simulink model "sl_subsys_fcncallerr12"  (Simulink 7.6)
settings: Solver=FixedStepDiscrete  StartTime=0.0  StopTime=10.0  FixedStep=1  RelTol=1e-3
libraries: simulink x4
Description:
  | Function-call subsystems whose inputs are directly or indirectly computed during execution of the function-call
  | 
  | In each of the function-call subsystems below, one of the inputs is either directly
  | or indirectly computed during the computation of the function-call subsystems outputs. As
  | a result, one can alter the output values produced by the function-call by subtly affecting the
  | execution order of blocks within the function call subsystem's outputs method.
  | 
  | For example, in the first example below, the output signals of the function-call subsystem
  | change if one changes the port number of the first Outport block to 2 and the port number
  | of the second Outport block to 1. A similar change in results can be observed in example 2. In
  | example 3, you may run into similar issues by altering when the second function-call subsystem
  | is executed within the context of the first function-call subsystem.
settings Model: Creator=The MathWorks Inc.  CovMetricSettings=d  ExtModeAutoUpdateStatusClock=off
settings DataIOCC: SignalLoggingName=logsOut
settings OptimizationCC: BlockReduction=off  BooleanDataType=off  InlineInvariantSignals=on  InitFltsAndDblsToZero=on  OptimizeModelRefInitCode=on  LifeSpan=1
settings DebuggingCC: SaveWithParameterizedLinksMsg=none  CheckExecutionContextPreStartOutputMsg=on  CheckExecutionContextRuntimeOutputMsg=on  SignalResolutionControl=TryResolveAllWithWarning  SolverPrmCheckMsg=none  MultiTaskDSMMsg=warning  MultiTaskCondExecSysMsg=none
settings ModelReferenceCC: UpdateModelReferenceTargets=IfOutOfDate
settings SFSimCC: SimParseCustomCode=off
settings RTWCC: SystemTargetFile=ert.tlc  TemplateMakefile=ert_default_tmf  Description=RTW Embedded Coder (no auto configuration)  GenerateReport=on  ProcessScript=ert_make_rtw_hook  IncludeHyperlinkInReport=on  LaunchReport=on  IncludeERTFirstTime=on
settings CodeAppCC: IgnoreCustomStorageClasses=off  CustomSymbolStrFcn=$F$N$M
settings ERTTargetCC: TargetFcnLib=ansi_tfl_tmw.mat  MultiwordLength=2048  GenerateSampleERTMain=on  SupportContinuousTime=on  SupportNonInlinedSFcns=on  ERTCustomFileTemplate=example_file_process.tlc  ConvertIfToSwitch=off

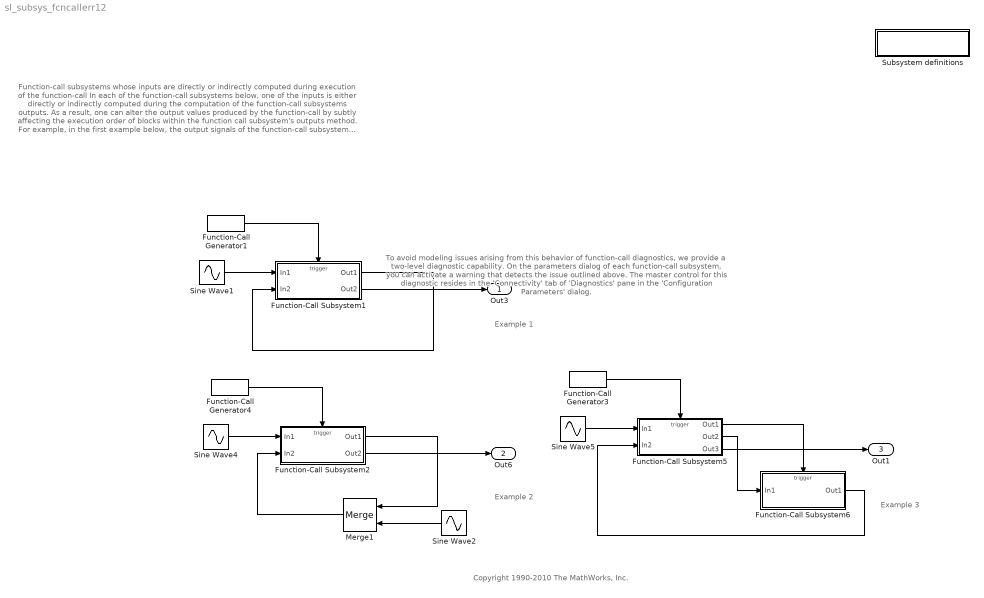
== system sl_subsys_fcncallerr12 ==
  note: Function-call subsystems whose inputs are directly or indirectly computed during
      | execution of the function-call
      |
      | In each of the function-call subsystems below, one of the inputs is either directly
      | or indirectly computed during the computation of the function-call subsystems outputs. As
      | a result, one can alter the output values produced by the function-call by subtly affecting the
      | execution order of blocks within the function call subsystem's outputs method.
      |
      | For example, in the first example below, the output signals of the function-call subsystem
      | change if one changes the port number of the first Outport block to 2 and the port number
      | of the second Outport block to 1. A similar change in results can be observed in example 2. In
      | example 3, you may run into similar issues by altering when the second function-call subsystem
      | is executed within the context of the first function-call subsystem.
  note: Example 1
  note: Example 2
  note: Example 3
  note: To avoid modeling issues arising from this behavior
      | of function-call diagnostics, we provide a two-level
      | diagnostic capability. On the parameters dialog of each
      | function-call subsystem, you can activate a warning
      | that detects the issue outlined above. The master
      | control for this diagnostic resides in the 'Connectivity'
      | tab of 'Diagnostics' pane in the 'Configuration Parameters'
      | dialog.
  note: Copyright 1990-2010 The MathWorks, Inc.
  " Subsystem definitions" : Subsystem
      settings: OpenFcn=helpview([matlabroot,'/toolbox/simulink/simdemos/simfeatures/html/sl_subsys_definitions.html']);
      mask Display: disp('Subsystem\ndefinitions')
  Function-Call Generator1 : simulink/Ports & Subsystems/Function-Call Generator  sample_time=1  numberOfIterations=1
  Function-Call Generator3 : simulink/Ports & Subsystems/Function-Call Generator  sample_time=1  numberOfIterations=1
  Function-Call Generator4 : simulink/Ports & Subsystems/Function-Call Generator  sample_time=1  numberOfIterations=1
  Function-Call Subsystem1 : Subsystem  TreatAsAtomicUnit=on  CheckFcnCallInpInsideContextMsg=on
  Function-Call Subsystem2 : Subsystem  TreatAsAtomicUnit=on  CheckFcnCallInpInsideContextMsg=on
  Function-Call Subsystem5 : Subsystem  TreatAsAtomicUnit=on  CheckFcnCallInpInsideContextMsg=on
  Function-Call Subsystem6 : Subsystem  TreatAsAtomicUnit=on
  Merge1 : Merge
  Sine Wave{1..2,4..5} (4 alike) : Sin  SampleTime=1
  Out3 : Outport
  Out6 : Outport  Port=2
  Out1 : Outport  Port=3
  wires:
  Function-Call Subsystem1/2(Out2) -> Out3/1
  Function-Call Generator1/1 -> Function-Call Subsystem1/Trigger
  Sine Wave1/1 -> Function-Call Subsystem1/1(In1)
  Function-Call Subsystem1/1(Out1) -> Function-Call Subsystem1/2(In2)
  Function-Call Subsystem2/2(Out2) -> Out6/1
  Function-Call Generator4/1 -> Function-Call Subsystem2/Trigger
  Sine Wave4/1 -> Function-Call Subsystem2/1(In1)
  Function-Call Subsystem2/1(Out1) -> Merge1/1
  Merge1/1 -> Function-Call Subsystem2/2(In2)
  Sine Wave2/1 -> Merge1/2
  Function-Call Generator3/1 -> Function-Call Subsystem5/Trigger
  Sine Wave5/1 -> Function-Call Subsystem5/1(In1)
  Function-Call Subsystem5/1(Out1) -> Function-Call Subsystem6/Trigger
  Function-Call Subsystem5/2(Out2) -> Function-Call Subsystem6/1(In1)
  Function-Call Subsystem6/1(Out1) -> Function-Call Subsystem5/2(In2)
  Function-Call Subsystem5/3(Out3) -> Out1/1

== system sl_subsys_fcncallerr12/ Subsystem definitions ==

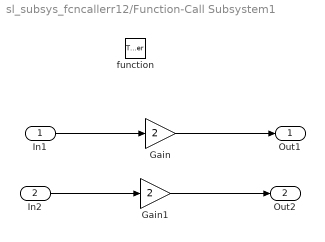
== system sl_subsys_fcncallerr12/Function-Call Subsystem1 ==
  In1 : Inport
  In2 : Inport  Port=2
  function : TriggerPort  TriggerType=function-call
  Gain : Gain  Gain=2
  Gain1 : Gain  Gain=2
  Out1 : Outport
  Out2 : Outport  Port=2
  wires:
  Gain1/1 -> Out2/1
  In2/1 -> Gain1/1
  Gain/1 -> Out1/1
  In1/1 -> Gain/1

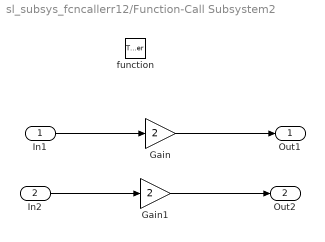
== system sl_subsys_fcncallerr12/Function-Call Subsystem2 ==
  In1 : Inport
  In2 : Inport  Port=2
  function : TriggerPort  TriggerType=function-call
  Gain : Gain  Gain=2
  Gain1 : Gain  Gain=2
  Out1 : Outport
  Out2 : Outport  Port=2
  wires:
  In1/1 -> Gain/1
  Gain/1 -> Out1/1
  In2/1 -> Gain1/1
  Gain1/1 -> Out2/1

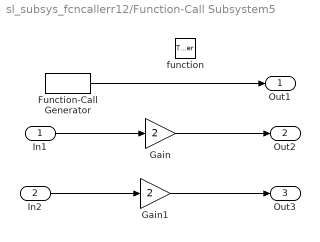
== system sl_subsys_fcncallerr12/Function-Call Subsystem5 ==
  In1 : Inport
  In2 : Inport  Port=2
  function : TriggerPort  TriggerType=function-call
  Function-Call Generator : simulink/Ports & Subsystems/Function-Call Generator  sample_time=-1  numberOfIterations=1
  Gain : Gain  Gain=2
  Gain1 : Gain  Gain=2
  Out1 : Outport
  Out2 : Outport  Port=2
  Out3 : Outport  Port=3
  wires:
  Function-Call Generator/1 -> Out1/1
  Gain1/1 -> Out3/1
  In2/1 -> Gain1/1
  Gain/1 -> Out2/1
  In1/1 -> Gain/1

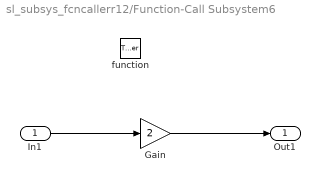
== system sl_subsys_fcncallerr12/Function-Call Subsystem6 ==
  In1 : Inport
  function : TriggerPort  TriggerType=function-call
  Gain : Gain  Gain=2
  Out1 : Outport
  wires:
  Gain/1 -> Out1/1
  In1/1 -> Gain/1
